simulink model "analiseLateroDirecional"  (R2016a)
settings: Solver=ode4  StartTime=0.0  StopTime=300  FixedStep=0.01  RelTol=1e-3
undefined symbols (not defined in the file): Cphi, degtorad, Kp, Kphi, Kpsi, Kr, tau
libraries: simulink x3, cstblocks x2
settings Model: Creator=IEE  LastModifiedBy=Marcelo
settings DataIOCC: LimitDataPoints=on  SaveFormat=Array
settings DebuggingCC: UnderspecifiedInitializationDetection=Classic  MergeDetectMultiDrivingBlocksExec=none  SolverPrmCheckMsg=warning  StateNameClashWarn=warning
settings HardwareCC: ProdBitPerPointer=32  ProdLargestAtomicFloat=None  ProdIntDivRoundTo=Undefined  ProdEndianess=Unspecified  ProdWordSize=32  ProdHWDeviceType=32-bit Generic
settings ModelReferenceCC: PropagateSignalLabelsOutOfModel=off
settings ConfigComp: CovModelRefEnable=Off

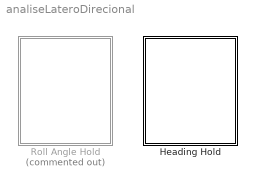
== system analiseLateroDirecional ==
  Heading Hold : Subsystem
  Roll Angle Hold : Subsystem  Commented=on

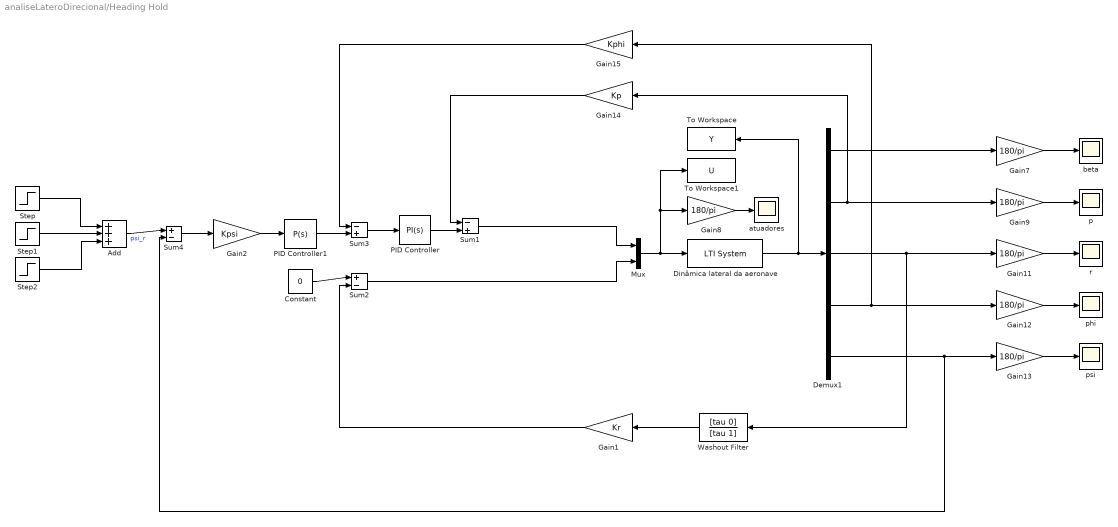
== system analiseLateroDirecional/Heading Hold ==
  Add : Sum  Inputs=+++
  Constant : Constant  Value=0
  Demux1 : Demux  Outputs=5
  Dinâmica lateral da aeronave : cstblocks/LTI System  sys=aeronave  IC=[]
  Gain1 : Gain  Gain=Kr
  Gain{7..9,11..13} (6 alike) : Gain  Gain=180/pi
  Gain14 : Gain  Gain=Kp
  Gain15 : Gain  Gain=Kphi
  Gain2 : Gain  Gain=Kpsi
  Mux : Mux  Inputs=2
  PID Controller : simulink/Continuous/PID Controller  Controller=PI  TimeDomain=Continuous-time  SampleTime=-1  IntegratorMethod=Forward Euler  FilterMethod=Forward Euler  Form=Parallel  UseFilter=on  ControllerParametersSource=internal  P=Cphi.Kp  I=Cphi.Ki  D=0  N=100  InitialConditionSource=internal  InitialConditionForIntegrator=0  InitialConditionForFilter=0  ExternalReset=none  LimitOutput=off  UpperSaturationLimit=inf  LowerSaturationLimit=-inf  LinearizeAsGain=on  AntiWindupMode=none  Kb=1  TrackingMode=off  Kt=1  PParamMin=[]  PParamMax=[]  IParamMin=[]  IParamMax=[]  DParamMin=[]  DParamMax=[]  NParamMin=[]  NParamMax=[]  KbParamMin=[]  KbParamMax=[]  KtParamMin=[]  KtParamMax=[]  POutMin=[]  POutMax=[]  IOutMin=[]  IOutMax=[]  DOutMin=[]  DOutMax=[]  NOutMin=[]  NOutMax=[]  KbOutMin=[]  KbOutMax=[]  KtOutMin=[]  KtOutMax=[]  IntegratorOutMin=[]  IntegratorOutMax=[]  FilterOutMin=[]  FilterOutMax=[]  SumOutMin=[]  SumOutMax=[]  SumI1OutMin=[]  SumI1OutMax=[]  SumI2OutMin=[]  SumI2OutMax=[]  SumI3OutMin=[]  SumI3OutMax=[]  SumDOutMin=[]  SumDOutMax=[]  SaturationOutMin=[]  SaturationOutMax=[]  IntegratorContinuousStateAttributes=''  IntegratorStateMustResolveToSignalObject=off  IntegratorRTWStateStorageClass=Auto  FilterContinuousStateAttributes=''  FilterStateMustResolveToSignalObject=off  FilterRTWStateStorageClass=Auto  DifferentiatorICPrevScaledInput=0  DifferentiatorOutMin=[]  DifferentiatorOutMax=[]
  PID Controller1 : simulink/Continuous/PID Controller  Controller=P  TimeDomain=Continuous-time  SampleTime=-1  IntegratorMethod=Forward Euler  FilterMethod=Forward Euler  Form=Parallel  UseFilter=on  ControllerParametersSource=internal  P=1  I=1  D=0  N=100  InitialConditionSource=internal  InitialConditionForIntegrator=0  InitialConditionForFilter=0  ExternalReset=none  LimitOutput=off  UpperSaturationLimit=inf  LowerSaturationLimit=-inf  LinearizeAsGain=on  AntiWindupMode=none  Kb=1  TrackingMode=off  Kt=1  PParamMin=[]  PParamMax=[]  IParamMin=[]  IParamMax=[]  DParamMin=[]  DParamMax=[]  NParamMin=[]  NParamMax=[]  KbParamMin=[]  KbParamMax=[]  KtParamMin=[]  KtParamMax=[]  POutMin=[]  POutMax=[]  IOutMin=[]  IOutMax=[]  DOutMin=[]  DOutMax=[]  NOutMin=[]  NOutMax=[]  KbOutMin=[]  KbOutMax=[]  KtOutMin=[]  KtOutMax=[]  IntegratorOutMin=[]  IntegratorOutMax=[]  FilterOutMin=[]  FilterOutMax=[]  SumOutMin=[]  SumOutMax=[]  SumI1OutMin=[]  SumI1OutMax=[]  SumI2OutMin=[]  SumI2OutMax=[]  SumI3OutMin=[]  SumI3OutMax=[]  SumDOutMin=[]  SumDOutMax=[]  SaturationOutMin=[]  SaturationOutMax=[]  IntegratorContinuousStateAttributes=''  IntegratorStateMustResolveToSignalObject=off  IntegratorRTWStateStorageClass=Auto  FilterContinuousStateAttributes=''  FilterStateMustResolveToSignalObject=off  FilterRTWStateStorageClass=Auto  DifferentiatorICPrevScaledInput=0  DifferentiatorOutMin=[]  DifferentiatorOutMax=[]
  Step : Step  Time=50  After=degtorad(45)  SampleTime=0
  Step1 : Step  Time=150  After=degtorad(-90)  SampleTime=0
  Step2 : Step  Time=250  After=degtorad(45)  SampleTime=0
  Sum1 : Sum  Inputs=|-+
  Sum2 : Sum  Inputs=|+-
  Sum3 : Sum  Inputs=|-+
  Sum4 : Sum  Inputs=|+-
  To Workspace : ToWorkspace  VariableName=Y  SaveFormat=Timeseries  SampleTime=-1
  To Workspace1 : ToWorkspace  VariableName=U  SaveFormat=Timeseries  SampleTime=-1
  Washout Filter : TransferFcn  Numerator=[tau 0]  Denominator=[tau 1]
  atuadores : Scope
  beta : Scope
  p : Scope
  phi : Scope
  psi : Scope
  r : Scope
  wires:
  Demux1/4 -> Gain15/1, Gain12/1
  Gain9/1 -> p/1
  Gain7/1 -> beta/1
  Demux1/2 -> Gain14/1, Gain9/1
  Gain12/1 -> phi/1
  Demux1/5 -> Sum4/2, Gain13/1
  Gain13/1 -> psi/1
  Gain11/1 -> r/1
  Demux1/1 -> Gain7/1
  Sum2/1 -> Mux/2
  Sum1/1 -> Mux/1
  PID Controller/1 -> Sum1/2
  Sum3/1 -> PID Controller/1
  Gain14/1 -> Sum1/1
  Gain15/1 -> Sum3/1
  Gain8/1 -> atuadores/1
  Dinâmica lateral da aeronave/1 -> To Workspace/1, Demux1/1
  Mux/1 -> Gain8/1, To Workspace1/1, Dinâmica lateral da aeronave/1
  Demux1/3 -> Washout Filter/1, Gain11/1
  Constant/1 -> Sum2/1
  Washout Filter/1 -> Gain1/1
  Gain1/1 -> Sum2/2
  Sum4/1 -> Gain2/1
  Step/1 -> Add/1
  Add/1 -> Sum4/1  "psi_r"
  Step1/1 -> Add/2
  Step2/1 -> Add/3
  PID Controller1/1 -> Sum3/2
  Gain2/1 -> PID Controller1/1

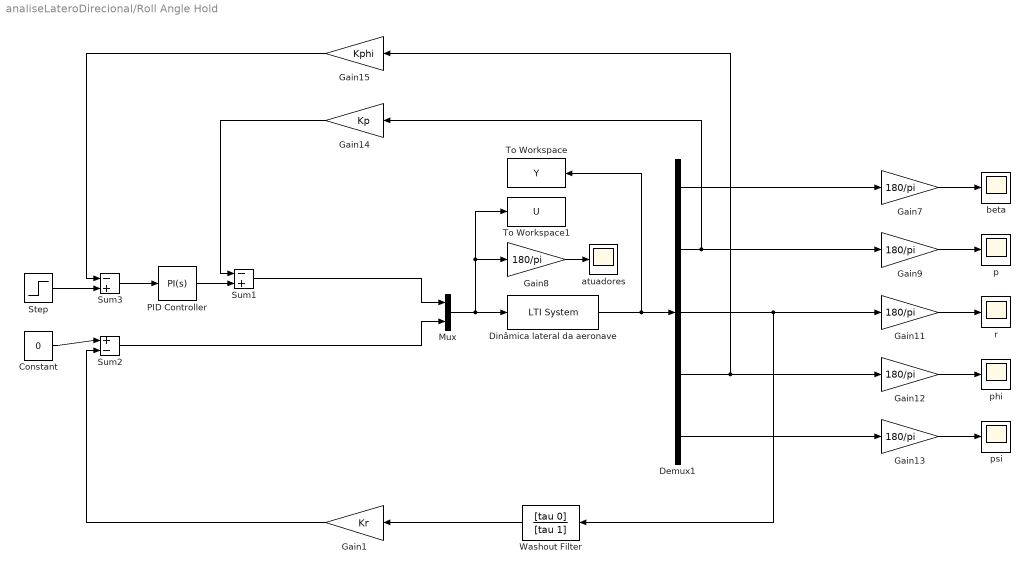
== system analiseLateroDirecional/Roll Angle Hold ==
  Constant : Constant  Value=0
  Demux1 : Demux  Outputs=5
  Dinâmica lateral da aeronave : cstblocks/LTI System  sys=aeronave  IC=[]
  Gain1 : Gain  Gain=Kr
  Gain{7..9,11..13} (6 alike) : Gain  Gain=180/pi
  Gain14 : Gain  Gain=Kp
  Gain15 : Gain  Gain=Kphi
  Mux : Mux  Inputs=2
  PID Controller : simulink/Continuous/PID Controller  Controller=PI  TimeDomain=Continuous-time  SampleTime=-1  IntegratorMethod=Forward Euler  FilterMethod=Forward Euler  Form=Parallel  UseFilter=on  ControllerParametersSource=internal  P=Cphi.Kp  I=Cphi.Ki  D=0  N=100  InitialConditionSource=internal  InitialConditionForIntegrator=0  InitialConditionForFilter=0  ExternalReset=none  LimitOutput=off  UpperSaturationLimit=inf  LowerSaturationLimit=-inf  LinearizeAsGain=on  AntiWindupMode=none  Kb=1  TrackingMode=off  Kt=1  PParamMin=[]  PParamMax=[]  IParamMin=[]  IParamMax=[]  DParamMin=[]  DParamMax=[]  NParamMin=[]  NParamMax=[]  KbParamMin=[]  KbParamMax=[]  KtParamMin=[]  KtParamMax=[]  POutMin=[]  POutMax=[]  IOutMin=[]  IOutMax=[]  DOutMin=[]  DOutMax=[]  NOutMin=[]  NOutMax=[]  KbOutMin=[]  KbOutMax=[]  KtOutMin=[]  KtOutMax=[]  IntegratorOutMin=[]  IntegratorOutMax=[]  FilterOutMin=[]  FilterOutMax=[]  SumOutMin=[]  SumOutMax=[]  SumI1OutMin=[]  SumI1OutMax=[]  SumI2OutMin=[]  SumI2OutMax=[]  SumI3OutMin=[]  SumI3OutMax=[]  SumDOutMin=[]  SumDOutMax=[]  SaturationOutMin=[]  SaturationOutMax=[]  IntegratorContinuousStateAttributes=''  IntegratorStateMustResolveToSignalObject=off  IntegratorRTWStateStorageClass=Auto  FilterContinuousStateAttributes=''  FilterStateMustResolveToSignalObject=off  FilterRTWStateStorageClass=Auto  DifferentiatorICPrevScaledInput=0  DifferentiatorOutMin=[]  DifferentiatorOutMax=[]
  Step : Step  Time=20  After=degtorad(20)  SampleTime=0
  Sum1 : Sum  Inputs=|-+
  Sum2 : Sum  Inputs=|+-
  Sum3 : Sum  Inputs=|-+
  To Workspace : ToWorkspace  VariableName=Y  SaveFormat=Timeseries  SampleTime=-1
  To Workspace1 : ToWorkspace  VariableName=U  SaveFormat=Timeseries  SampleTime=-1
  Washout Filter : TransferFcn  Numerator=[tau 0]  Denominator=[tau 1]
  atuadores : Scope
  beta : Scope
  p : Scope
  phi : Scope
  psi : Scope
  r : Scope
  wires:
  Demux1/4 -> Gain15/1, Gain12/1
  Gain9/1 -> p/1
  Gain7/1 -> beta/1
  Demux1/2 -> Gain14/1, Gain9/1
  Gain12/1 -> phi/1
  Demux1/5 -> Gain13/1
  Gain13/1 -> psi/1
  Gain11/1 -> r/1
  Demux1/1 -> Gain7/1
  Sum2/1 -> Mux/2
  Sum1/1 -> Mux/1
  PID Controller/1 -> Sum1/2
  Sum3/1 -> PID Controller/1
  Gain14/1 -> Sum1/1
  Gain15/1 -> Sum3/1
  Gain8/1 -> atuadores/1
  Dinâmica lateral da aeronave/1 -> To Workspace/1, Demux1/1
  Mux/1 -> Gain8/1, To Workspace1/1, Dinâmica lateral da aeronave/1
  Demux1/3 -> Washout Filter/1, Gain11/1
  Constant/1 -> Sum2/1
  Washout Filter/1 -> Gain1/1
  Gain1/1 -> Sum2/2
  Step/1 -> Sum3/2
